simulink model "Team2_PowerLine_Model_v03"  (R2026a)
settings: Solver=VariableStepAuto  StopTime=0.1  MaxStep=1e-4
libraries: simulink x2
settings Model: Creator=ruyxv  LastModifiedBy=ruyxv

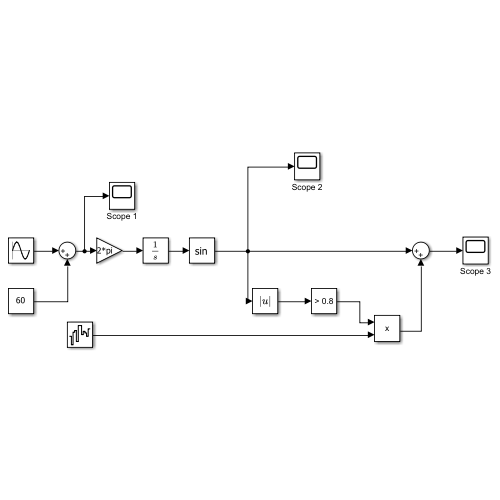
[thumbnail: Simulink's stored preview of the top-level diagram]
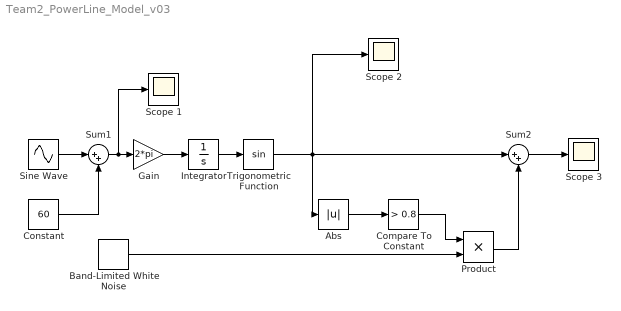
== system Team2_PowerLine_Model_v03 ==
  Abs : Abs  SaturateOnIntegerOverflow=off
  Band-Limited White Noise : simulink/Sources/Band-Limited White Noise  Cov=1e-5  Ts=1e-4  seed=[23341]
  Compare To Constant : simulink/Logic and Bit Operations/Compare To Constant  relop=>  const=0.8  OutDataTypeStr=boolean
  Constant : Constant  Value=60
  Gain : Gain  Gain=2*pi
  Integrator : Integrator
  Product : Product
  Scope 1 : Scope
      settings: ActiveDisplayYMinimum=59.975000000035017  ActiveDisplayYMaximum=60.02499999996499
  Scope 2 : Scope
      settings: ActiveDisplayYMinimum=-1  ActiveDisplayYMaximum=1
  Scope 3 : Scope
      settings: ActiveDisplayYMinimum=-2.2103679570534909  ActiveDisplayYMaximum=2.1818220916576165  DataLoggingVariableName=ScopeData2
  Sine Wave : Sin  Amplitude=0.02  Frequency=2*pi*0.5  SampleTime=0
  Sum1 : Sum  Inputs=|++
  Sum2 : Sum  Inputs=|++
  Trigonometric Function : Trigonometry
  wires:
  Sine Wave/1 -> Sum1/1
  Gain/1 -> Integrator/1
  Constant/1 -> Sum1/2
  Sum1/1 -> Scope 1/1, Gain/1
  Integrator/1 -> Trigonometric Function/1
  Abs/1 -> Compare To Constant/1
  Compare To Constant/1 -> Product/1
  Band-Limited White Noise/1 -> Product/2
  Sum2/1 -> Scope 3/1
  Product/1 -> Sum2/2
  Trigonometric Function/1 -> Abs/1, Scope 2/1, Sum2/1
